simulink model "RP_ROS_Stateflow"  (R2022a)
settings: Solver=ode23t  StartTime=0.0  StopTime=inf  RelTol=1e-3
InitFcn:
  | RPInit
  | set_param([gcs '/RP ROS Robot/Enabled'],'Value','1')
  | RP_ROS2_srv_eStop
model workspace (MAT data in the model file):
  mapForSim : object (value not decoded)
  occGrid : robotics.BinaryOccupancyGrid (value not decoded)
undefined symbols (not defined in the file): FloorSurface, Ref, RobotSurface, X, Y, Z
libraries: sm_lib x21, ros2lib x15, RP_Simulator_Components x15, nesl_utility x11, RoboticsPlayground x5
(part 2 of 2)

== system RP_ROS_Stateflow/RP ROS Robot/Obstacle Environment/Robot/Sensor Visuals ==
  US Visual1 : RP_Simulator_Components/US Visual  size=1  color=[0.5 0.1 0.1]  pose=[0.25 0]  angle=0
  US Visual2 : RP_Simulator_Components/US Visual  size=1  color=[0.5 0.1 0.1]  pose=[0.15 0.15]  angle=90
  US Visual3 : RP_Simulator_Components/US Visual  size=1  color=[0.5 0.1 0.1]  pose=[0.15 -0.15]  angle=-90
  Robot : PMIOPort  Side=Left
  connections:
  US Visual1/LConn1 -- Robot/RConn1 -- US Visual2/LConn1 -- US Visual3/LConn1

== stateflow chart RP_ROS_Stateflow/Navigate Maze ==
  state TurnLeft
    LeftMotor=-100;
    RightMotor=100;
  state TurnRight
    LeftMotor=100;
    RightMotor=-100;
  state MoveForward
    LeftMotor=100;
    RightMotor=100;
  (default) -> MoveForward
  MoveForward -> TurnLeft [order 2] : [frontDist < 0.6 && rightDist < 1]
  MoveForward -> TurnRight [order 1] : [frontDist < 0.6 && leftDist < 1]
  TurnRight -> MoveForward : [after(2,sec)]
  TurnLeft -> MoveForward : [after(2,sec)]
  data: LeftMotor output; RightMotor output; frontDist input; leftDist input; rightDist input
